simulink subsystem "referenceSigs"  (R2025b)
settings: Solver=VariableStepAuto  StartTime=0.0  StopTime=10.0  RelTol=1e-3
values from neighbouring files (symbols this model uses):
  stepTime = 10    [FOSWECparameters.m]
  T = 5    [FOSWECparameters.m]
  Ts = 0.001    [FOSWECparameters.m]
undefined symbols (not defined in the file or in its folder): Tsin
libraries: simulink x15, dspsrcs4 x1
settings Model: Creator=bosmab  LastModifiedBy=bosmab

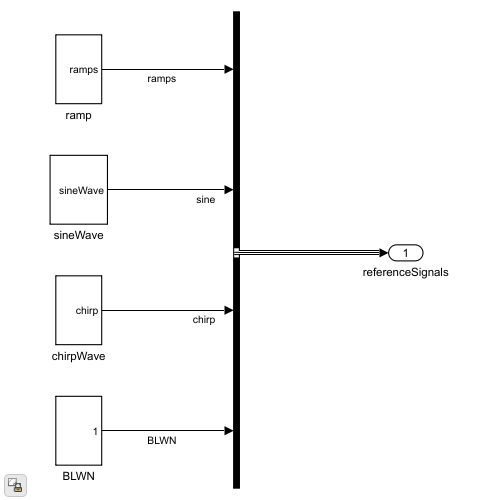
[thumbnail: Simulink's stored preview of the top-level diagram]
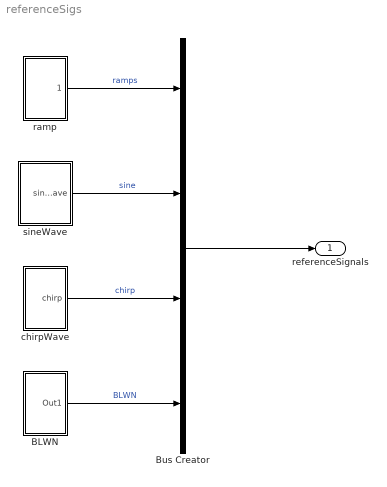
== system referenceSigs ==
  BLWN : Subsystem
  Bus Creator : BusCreator  Inputs=4
  chirpWave : Subsystem
  ramp : Subsystem
  sineWave : Subsystem
  referenceSignals : Outport
  wires:
  Bus Creator/1 -> referenceSignals/1
  chirpWave/1(chirp) -> Bus Creator/3  "chirp"
  ramp/1(ramps) -> Bus Creator/1  "ramps"
  sineWave/1(sineWave) -> Bus Creator/2  "sine"
  BLWN/1(Out1) -> Bus Creator/4  "BLWN"

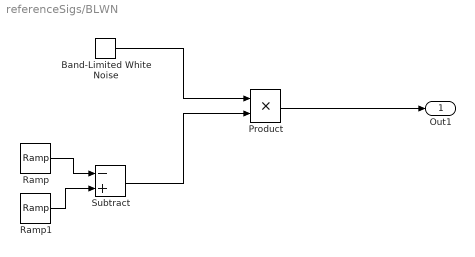
== system referenceSigs/BLWN ==
  Band-Limited White Noise : simulink/Sources/Band-Limited White Noise  Cov=[0.0001]  Ts=Ts  seed=[23341]
  Product : Product
  Ramp : simulink/Sources/Ramp  slope=1/(5*T)  start=stepTime  InitialOutput=0
  Ramp1 : simulink/Sources/Ramp  slope=1/(5*T)  start=stepTime+5*T  InitialOutput=0
  Subtract : Sum  Inputs=-+
  Out1 : Outport  OutDataTypeStr=double  PortDimensions=1  SampleTime=0
  wires:
  Band-Limited White Noise/1 -> Product/1
  Product/1 -> Out1/1
  Ramp/1 -> Subtract/1
  Subtract/1 -> Product/2
  Ramp1/1 -> Subtract/2

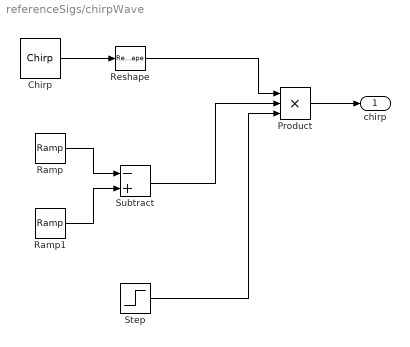
== system referenceSigs/chirpWave ==
  Chirp : dspsrcs4/Chirp  sweep=Linear  mode=Unidirectional  f0=.1  f1=1  t1=300  Tsweep=300  phase=0  Ts=1/1000  spf=1  datatype=double  OutputFrames=off
  Product : Product  Inputs=3
  Ramp : simulink/Sources/Ramp  slope=1/(5*T)  start=2*stepTime  InitialOutput=0
  Ramp1 : simulink/Sources/Ramp  slope=1/(5*T)  start=2*stepTime+5*T  InitialOutput=0
  Reshape : Reshape
  Step : Step  Time=stepTime  SampleTime=0
  Subtract : Sum  Inputs=-+
  chirp : Outport
  wires:
  Product/1 -> chirp/1
  Reshape/1 -> Product/1
  Step/1 -> Product/3
  Subtract/1 -> Product/2
  Chirp/1 -> Reshape/1
  Ramp/1 -> Subtract/1
  Ramp1/1 -> Subtract/2

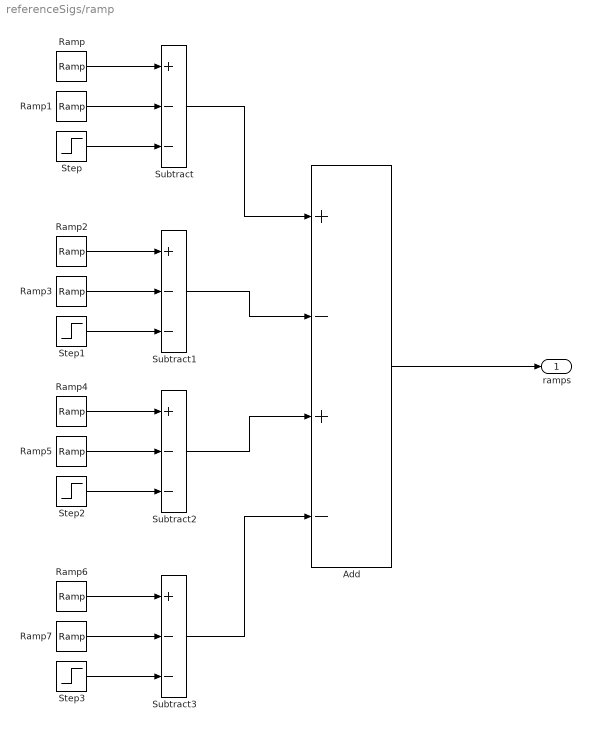
== system referenceSigs/ramp ==
  Add : Sum  Inputs=+-+-
  Ramp : simulink/Sources/Ramp  slope=1/(t(2)-t(1))  start=t(1)  InitialOutput=0
  Ramp1 : simulink/Sources/Ramp  slope=1/(t(2)-t(1))  start=t(2)  InitialOutput=0
  Ramp2 : simulink/Sources/Ramp  slope=1/(t(4)-t(3))  start=t(3)  InitialOutput=0
  Ramp3 : simulink/Sources/Ramp  slope=1/(t(4)-t(3))  start=t(4)  InitialOutput=0
  Ramp4 : simulink/Sources/Ramp  slope=1/(t(6)-t(5))  start=t(5)  InitialOutput=0
  Ramp5 : simulink/Sources/Ramp  slope=1/(t(6)-t(5))  start=t(6)  InitialOutput=0
  Ramp6 : simulink/Sources/Ramp  slope=1/(t(8)-t(7))  start=t(7)  InitialOutput=0
  Ramp7 : simulink/Sources/Ramp  slope=1/(t(8)-t(7))  start=t(8)  InitialOutput=0
  Step : Step  Time=t(2)  SampleTime=0
  Step1 : Step  Time=t(4)  SampleTime=0
  Step2 : Step  Time=t(6)  SampleTime=0
  Step3 : Step  Time=t(8)  SampleTime=0
  Subtract{,1..3} (4 alike) : Sum  Inputs=+--
  ramps : Outport  OutDataTypeStr=double  PortDimensions=1  SampleTime=0
  wires:
  Ramp7/1 -> Subtract3/2
  Step3/1 -> Subtract3/3
  Ramp1/1 -> Subtract/2
  Ramp4/1 -> Subtract2/1
  Step2/1 -> Subtract2/3
  Step/1 -> Subtract/3
  Subtract2/1 -> Add/3
  Subtract/1 -> Add/1
  Ramp6/1 -> Subtract3/1
  Ramp2/1 -> Subtract1/1
  Ramp3/1 -> Subtract1/2
  Subtract3/1 -> Add/4
  Step1/1 -> Subtract1/3
  Ramp/1 -> Subtract/1
  Ramp5/1 -> Subtract2/2
  Subtract1/1 -> Add/2
  Add/1 -> ramps/1

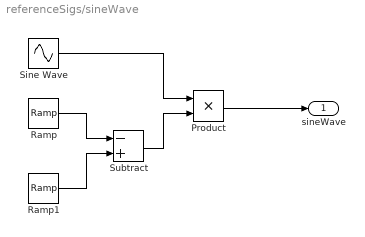
== system referenceSigs/sineWave ==
  Product : Product
  Ramp : simulink/Sources/Ramp  slope=1/(5*T)  start=stepTime  InitialOutput=0
  Ramp1 : simulink/Sources/Ramp  slope=1/(5*T)  start=stepTime+5*T  InitialOutput=0
  Sine Wave : Sin  Frequency=2*pi/Tsin  SampleTime=0
  Subtract : Sum  Inputs=-+
  sineWave : Outport  OutDataTypeStr=double  PortDimensions=1  SampleTime=0
  wires:
  Ramp1/1 -> Subtract/2
  Subtract/1 -> Product/2
  Sine Wave/1 -> Product/1
  Ramp/1 -> Subtract/1
  Product/1 -> sineWave/1
